simulink model "HSat_orbit"  (R2023a)
settings: Solver=FixedStepAuto  StartTime=0  StopTime=86400*900  MaxStep=3600  RelTol=1e-3  EnableMultiTasking=on
values from neighbouring files (symbols this model uses):
  ext_ENV_G = 6.674e-11    [HSat_op_setup.m]    (also in HSat_op_setup_merged_maria.m)
  ext_ENV_muEarth = 3.986005e14    (= 398600500000000)    [GEO_insertion_setup.m]    (also in HSat_op_setup.m; HSat_op_setup_merged_maria.m; init_orbit_analysis_with_drag_loss.m)
  ext_ENV_Re = 6.37813700*10^6    (= 6378137)    [HSat_op_setup.m]    (also in HSat_op_setup_merged_maria.m)
  ext_EOR_atmosphere_end = 1000e3    (= 1000000)    [HSat_op_setup.m]    (also in HSat_op_setup_merged_maria.m)
  ext_EOR_perigeeraise_end = 600e3    (= 600000)    [HSat_op_setup.m]    (also in HSat_op_setup_merged_maria.m)
  ext_Main_initDate_IC_T = sim_start    [HSat_op_setup.m]    (also in HSat_op_setup_merged_maria.m)
  ext_SC_activecorr_COE_ECI = [1, 1, 1, 0, 0, 0, 0, 0 ]    [HSat_op_setup.m]    (also in HSat_op_setup_merged_maria.m)
  ext_SC_balanced_COE_ECI = [ .500    0.70    1.100 1 1]    [HSat_op_setup.m]    (also in HSat_op_setup_merged_maria.m = [ 0.10 2.10 1.40    1.0000    1.0000]; launch_settings.m)
  ext_SC_cutofferror_COE_ECI = [150e3, .01, 0.1*pi/180, .1*pi/180,.1*pi/180, 0, 0, 0]    [HSat_op_setup.m]    (also in HSat_op_setup_merged_maria.m)
  ext_SC_init_COE_ECI = [a0,ecc0,i0,an0,ap0,tran0,eccan0,ma0]    [HSat_op_setup.m]    (also in HSat_op_setup_merged_maria.m)
  ext_SC_target_COE_ECI = [a1,ecc1,i1,an1,ap1,tran1,eccan1,ma1]    [HSat_op_setup.m]    (also in HSat_op_setup_merged_maria.m)
  ext_SC_target_lambda = 67*pi/180    (= 1.16937059884)    [HSat_op_setup.m]    (also in HSat_op_setup_merged_maria.m)
  sim_SC_init_CoG_EOR_dry = [-0.00448 0.00106 0.46931]    [HSat_op_setup.m]    (also in HSat_op_setup_merged_maria.m)
  sim_SC_init_CoG_propellant = [0 0 0.24758]    [HSat_op_setup.m]    (also in HSat_op_setup_merged_maria.m)
  sim_SC_init_dry_mass = sim_SC_init_wet_mass-sim_SC_init_propellant_mass    (= 727)    [HSat_op_setup.m]    (also in HSat_op_setup_merged_maria.m = 813.7)
  sim_SC_init_wet_mass = 750    [HSat_op_setup.m]    (also in HSat_op_setup_merged_maria.m)
  sim_thrust_force = [ ... (first row only)    [HSat_op_setup.m]    (also in HSat_op_setup_merged_maria.m)
  sim_thrust_massflow = [ ... (first row only)    [HSat_op_setup.m]    (also in HSat_op_setup_merged_maria.m)
  sim_thrust_vector = [ ... (first row only)    [HSat_op_setup.m]    (also in HSat_op_setup_merged_maria.m)
  sim_thruster_position = [ ... (first row only)    [HSat_op_setup.m]    (also in HSat_op_setup_merged_maria.m)
  sim_ts_save = 60    [HSat_op_setup.m]    (also in HSat_op_setup_merged_maria.m)
  third_body_jupiter = 1    [HSat_op_setup.m]    (also in HSat_op_setup_merged_maria.m)
  third_body_moon = 1    [HSat_op_setup.m]    (also in HSat_op_setup_merged_maria.m)
  third_body_sun = 1    [HSat_op_setup.m]    (also in HSat_op_setup_merged_maria.m)
libraries: aerolibutil x26, simulink x12, sharedtransform x7, sharedutil x4, Toolbox x3, matrix_library x1, simulink_extras x1
(part 3 of 5)

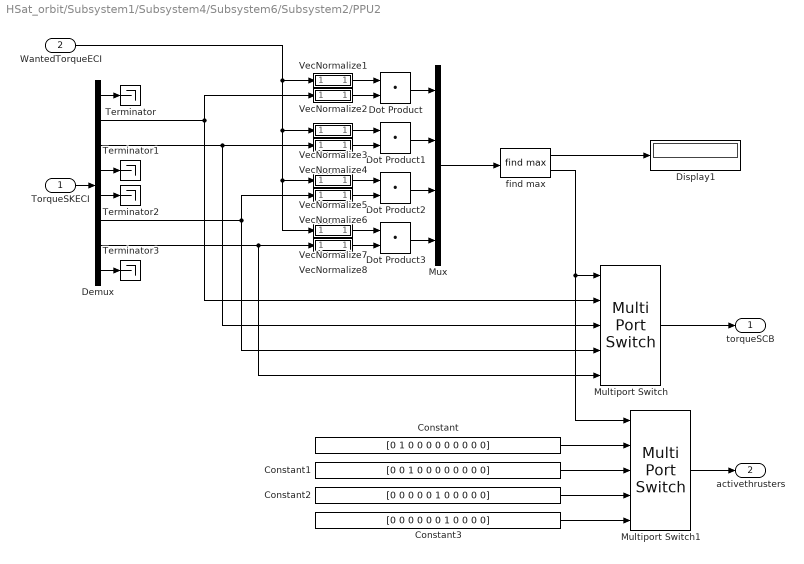
== system HSat_orbit/Subsystem1/Subsystem4/Subsystem6/Subsystem2/PPU2 ==
  TorqueSKECI : Inport
  WantedTorqueECI : Inport  Port=2
  Constant : Constant  Value=[0 1 0 0 0 0 0 0 0 0 0]
  Constant1 : Constant  Value=[0 0 1 0 0 0 0 0 0 0 0]
  Constant2 : Constant  Value=[0 0 0 0 0 1 0 0 0 0 0]
  Constant3 : Constant  Value=[0 0 0 0 0 0 1 0 0 0 0]
  Demux : Demux  Outputs=8
  Display1 : Display
  Dot Product{,1..3} (4 alike) : DotProduct  OutDataTypeStr=Inherit: Inherit via internal rule
  Multiport Switch : MultiPortSwitch  Inputs=4  SaturateOnIntegerOverflow=off  InputSameDT=off
  Multiport Switch1 : MultiPortSwitch  Inputs=4  SaturateOnIntegerOverflow=off  InputSameDT=off
  Mux : Mux
  Terminator{,1..3} (4 alike) : Terminator
  VecNormalize1 : Subsystem
      mask Display: disp('u/||u||')
  VecNormalize2 : Subsystem
      mask Display: disp('u/||u||')
  VecNormalize3 : Subsystem
      mask Display: disp('u/||u||')
  VecNormalize4 : Subsystem
      mask Display: disp('u/||u||')
  VecNormalize5 : Subsystem
      mask Display: disp('u/||u||')
  VecNormalize6 : Subsystem
      mask Display: disp('u/||u||')
  VecNormalize7 : Subsystem
      mask Display: disp('u/||u||')
  VecNormalize8 : Subsystem
      mask Display: disp('u/||u||')
  find max : Toolbox/vector blocks/find max  SystemSampleTime=-1  VariantActivationTime=update diagram  Latency=0  AutoFrameSizeCalculation=off
      settings: SourceProductName=SSC flight toolbox
  torqueSCB : Outport
  activethrusters : Outport  Port=2
  wires:
  TorqueSKECI/1 -> Demux/1
  Demux/2 -> VecNormalize2/1(In1), Multiport Switch/2
  Demux/3 -> Multiport Switch/3, VecNormalize4/1(In1)
  Demux/6 -> VecNormalize6/1(In1), Multiport Switch/4
  Demux/7 -> Multiport Switch/5, VecNormalize8/1(In1)
  WantedTorqueECI/1 -> VecNormalize1/1(In1), VecNormalize3/1(In1), VecNormalize5/1(In1), VecNormalize7/1(In1)
  VecNormalize1/1(Out1) -> Dot Product/1
  VecNormalize2/1(Out1) -> Dot Product/2
  VecNormalize3/1(Out1) -> Dot Product1/1
  VecNormalize4/1(Out1) -> Dot Product1/2
  VecNormalize5/1(Out1) -> Dot Product2/1
  VecNormalize6/1(Out1) -> Dot Product2/2
  VecNormalize7/1(Out1) -> Dot Product3/1
  VecNormalize8/1(Out1) -> Dot Product3/2
  Dot Product/1 -> Mux/1
  Dot Product1/1 -> Mux/2
  Dot Product2/1 -> Mux/3
  Dot Product3/1 -> Mux/4
  Mux/1 -> find max/1
  find max/1 -> Display1/1
  Multiport Switch/1 -> torqueSCB/1
  Demux/5 -> Terminator2/1
  Demux/4 -> Terminator1/1
  Demux/1 -> Terminator/1
  Demux/8 -> Terminator3/1
  Multiport Switch1/1 -> activethrusters/1
  Constant/1 -> Multiport Switch1/2
  Constant1/1 -> Multiport Switch1/3
  Constant3/1 -> Multiport Switch1/5
  find max/2 -> Multiport Switch1/1, Multiport Switch/1
  Constant2/1 -> Multiport Switch1/4

== system HSat_orbit/Subsystem1/Subsystem4/Subsystem6/Subsystem2/Subsystem ==
  AllTorquesSCB : Inport
  q_eci2scb_wanted : Inport  Port=2
  Mux : Mux  Inputs=8
  Quaternion Rotation{,1..7} (8 alike) : aerolibutil/Quaternion Rotation
  TorqueSCBSK1 : Selector  NumberOfDimensions=2  InputPortWidth=3  IndexOptions=Index vector (dialog),Index vector (dialog)  Indices=1,[1 2 3]  OutputSizes=1,1
  TorqueSCBSK2 : Selector  NumberOfDimensions=2  InputPortWidth=3  IndexOptions=Index vector (dialog),Index vector (dialog)  Indices=2,[1 2 3]  OutputSizes=1,1
  TorqueSCBSK3 : Selector  NumberOfDimensions=2  InputPortWidth=3  IndexOptions=Index vector (dialog),Index vector (dialog)  Indices=3,[1 2 3]  OutputSizes=1,1
  TorqueSCBSK4 : Selector  NumberOfDimensions=2  InputPortWidth=3  IndexOptions=Index vector (dialog),Index vector (dialog)  Indices=4,[1 2 3]  OutputSizes=1,1
  TorqueSCBSK5 : Selector  NumberOfDimensions=2  InputPortWidth=3  IndexOptions=Index vector (dialog),Index vector (dialog)  Indices=5,[1 2 3]  OutputSizes=1,1
  TorqueSCBSK6 : Selector  NumberOfDimensions=2  InputPortWidth=3  IndexOptions=Index vector (dialog),Index vector (dialog)  Indices=6,[1 2 3]  OutputSizes=1,1
  TorqueSCBSK7 : Selector  NumberOfDimensions=2  InputPortWidth=3  IndexOptions=Index vector (dialog),Index vector (dialog)  Indices=7,[1 2 3]  OutputSizes=1,1
  TorqueSCBSK8 : Selector  NumberOfDimensions=2  InputPortWidth=3  IndexOptions=Index vector (dialog),Index vector (dialog)  Indices=8,[1 2 3]  OutputSizes=1,1
  TorqueSKECI : Outport
  wires:
  TorqueSCBSK5/1 -> Quaternion Rotation4/2
  Quaternion Rotation3/1 -> Mux/4  "TorqueECISK4"
  Quaternion Rotation6/1 -> Mux/7  "TorqueECISK7"
  Quaternion Rotation4/1 -> Mux/5  "TorqueECISK5"
  TorqueSCBSK3/1 -> Quaternion Rotation2/2
  Quaternion Rotation/1 -> Mux/1  "TorqueECISK1"
  Quaternion Rotation7/1 -> Mux/8  "TorqueECISK8"
  TorqueSCBSK2/1 -> Quaternion Rotation1/2
  Quaternion Rotation2/1 -> Mux/3  "TorqueECISK3"
  TorqueSCBSK4/1 -> Quaternion Rotation3/2
  q_eci2scb_wanted/1 -> Quaternion Rotation7/1, Quaternion Rotation6/1, Quaternion Rotation5/1, Quaternion Rotation4/1, Quaternion Rotation3/1, Quaternion Rotation2/1, Quaternion Rotation1/1, Quaternion Rotation/1
  TorqueSCBSK8/1 -> Quaternion Rotation7/2
  TorqueSCBSK7/1 -> Quaternion Rotation6/2
  TorqueSCBSK1/1 -> Quaternion Rotation/2
  Quaternion Rotation5/1 -> Mux/6  "TorqueECISK6"
  TorqueSCBSK6/1 -> Quaternion Rotation5/2
  AllTorquesSCB/1 -> TorqueSCBSK8/1, TorqueSCBSK7/1, TorqueSCBSK6/1, TorqueSCBSK5/1, TorqueSCBSK4/1, TorqueSCBSK3/1, TorqueSCBSK2/1, TorqueSCBSK1/1
  Quaternion Rotation1/1 -> Mux/2  "TorqueECISK2"
  Mux/1 -> TorqueSKECI/1

== system HSat_orbit/Subsystem1/Subsystem4/Subsystem6/Subsystem2/Subsystem1 ==
  TorqueSCB : Inport
  WantedTorqueECI : Inport  Port=2
  sunvECI : Inport  Port=3
  Quaternion Multiplication : aerolibutil/Quaternion Multiplication
  Subsystem : Subsystem
  q_scb_calc : Subsystem
  q_eci2scb : Outport
  wires:
  Quaternion Multiplication/1 -> q_eci2scb/1
  sunvECI/1 -> q_scb_calc/2(sunvECI)
  q_scb_calc/1(qECI2scbp) -> Quaternion Multiplication/1
  TorqueSCB/1 -> Subsystem/1(EORthrustSCB)
  Subsystem/1(qscbp2scb) -> Quaternion Multiplication/2
  WantedTorqueECI/1 -> q_scb_calc/1(torqueECI)  "vec_eci"

== system HSat_orbit/Subsystem1/Dynamics/Subsystem/3 body perturbation legendre polynomial/Subsystem1/cos angle ==
  sat : Inport
  3 body : Inport  Port=2
  Divide : Product  Inputs=*//
  Dot Product : DotProduct  OutDataTypeStr=Inherit: Inherit via internal rule
  Dot Product1 : DotProduct  OutDataTypeStr=Inherit: Inherit via internal rule
  Dot Product2 : DotProduct  OutDataTypeStr=Inherit: Inherit via internal rule
  Sqrt : Sqrt
  Sqrt1 : Sqrt
  cos angle : Outport
  wires:
  3 body/1 -> Dot Product1/2, Dot Product1/1, Dot Product/2
  Dot Product1/1 -> Sqrt/1
  sat/1 -> Dot Product/1, Dot Product2/1, Dot Product2/2
  Dot Product2/1 -> Sqrt1/1
  Dot Product/1 -> Divide/1
  Sqrt/1 -> Divide/3
  Sqrt1/1 -> Divide/2
  Divide/1 -> cos angle/1

== system HSat_orbit/Subsystem1/Dynamics/Subsystem/3 body perturbation legendre polynomial/Subsystem2/cos angle ==
  sat : Inport
  3 body : Inport  Port=2
  Divide : Product  Inputs=*//
  Dot Product : DotProduct  OutDataTypeStr=Inherit: Inherit via internal rule
  Dot Product1 : DotProduct  OutDataTypeStr=Inherit: Inherit via internal rule
  Dot Product2 : DotProduct  OutDataTypeStr=Inherit: Inherit via internal rule
  Sqrt : Sqrt
  Sqrt1 : Sqrt
  cos angle : Outport
  wires:
  3 body/1 -> Dot Product1/2, Dot Product1/1, Dot Product/2
  Dot Product1/1 -> Sqrt/1
  sat/1 -> Dot Product/1, Dot Product2/1, Dot Product2/2
  Dot Product2/1 -> Sqrt1/1
  Dot Product/1 -> Divide/1
  Sqrt/1 -> Divide/3
  Sqrt1/1 -> Divide/2
  Divide/1 -> cos angle/1

== system HSat_orbit/Subsystem1/Dynamics/Subsystem/3 body perturbation legendre polynomial/Subsystem3/cos angle ==
  sat : Inport
  3 body : Inport  Port=2
  Divide : Product  Inputs=*//
  Dot Product : DotProduct  OutDataTypeStr=Inherit: Inherit via internal rule
  Dot Product1 : DotProduct  OutDataTypeStr=Inherit: Inherit via internal rule
  Dot Product2 : DotProduct  OutDataTypeStr=Inherit: Inherit via internal rule
  Sqrt : Sqrt
  Sqrt1 : Sqrt
  cos angle : Outport
  wires:
  3 body/1 -> Dot Product1/2, Dot Product1/1, Dot Product/2
  Dot Product1/1 -> Sqrt/1
  sat/1 -> Dot Product/1, Dot Product2/1, Dot Product2/2
  Dot Product2/1 -> Sqrt1/1
  Dot Product/1 -> Divide/1
  Sqrt/1 -> Divide/3
  Sqrt1/1 -> Divide/2
  Divide/1 -> cos angle/1

== system HSat_orbit/Subsystem1/Navigation/Subsystem/Subsystem2/Subsystem1/Norm3 ==
  In1 : Inport
  Dot Product : DotProduct  OutDataTypeStr=Inherit: Inherit via internal rule
  Sqrt : Sqrt
  Out1 : Outport
  wires:
  In1/1 -> Dot Product/1, Dot Product/2
  Sqrt/1 -> Out1/1
  Dot Product/1 -> Sqrt/1

== system HSat_orbit/Subsystem1/Navigation/Subsystem/Subsystem2/Subsystem1/Subsystem ==
  lambda : Inport
  Constant2 : Constant  Value=2*pi
  Constant3 : Constant  Value=pi
  Math Function2 : Math  Operator=mod
  Sum10 : Sum  Inputs=|+-
  Sum9 : Sum  Inputs=|++
  Out1 : Outport
  wires:
  lambda/1 -> Sum9/1
  Sum9/1 -> Math Function2/1
  Constant3/1 -> Sum9/2, Sum10/2
  Math Function2/1 -> Sum10/1
  Sum10/1 -> Out1/1
  Constant2/1 -> Math Function2/2

== system HSat_orbit/Subsystem1/Navigation/Subsystem/Subsystem2/Subsystem1/Subsystem1 ==
  lambda : Inport
  Constant4 : Constant  Value=2*pi
  Constant5 : Constant  Value=pi
  Math Function3 : Math  Operator=mod
  Sum11 : Sum  Inputs=|+-
  Sum12 : Sum  Inputs=|++
  Out1 : Outport
  wires:
  Sum11/1 -> Out1/1
  lambda/1 -> Sum12/1
  Sum12/1 -> Math Function3/1
  Math Function3/1 -> Sum11/1
  Constant5/1 -> Sum12/2, Sum11/2
  Constant4/1 -> Math Function3/2

== system HSat_orbit/Subsystem1/Navigation/Subsystem/Subsystem2/Subsystem1/Subsystem2 ==
  a : Inport
  Constant1 : Constant  Value=ext_ENV_muEarth
  Constant2 : Constant  Value=3
  Constant4 : Constant
  Divide : Product  Inputs=*/
  Gain : Gain  Gain=2*pi
  Gain1 : Gain  Gain=2*pi
  Gain3 : Gain
  Gain4 : Gain  Gain=1/86400
  Math Function : Math  Operator=pow
  Math Function1 : Math  Operator=reciprocal
  Sqrt : Sqrt
  Subtract : Sum  Inputs=+-
  lambdadot : Outport
  wires:
  Subtract/1 -> Gain1/1  "lambdadot"
  Constant4/1 -> Subtract/2
  Constant2/1 -> Math Function/2
  Sqrt/1 -> Gain/1
  Math Function/1 -> Divide/1
  Constant1/1 -> Divide/2
  Math Function1/1 -> Gain3/1
  a/1 -> Math Function/1
  Divide/1 -> Sqrt/1
  Gain1/1 -> lambdadot/1
  Gain/1 -> Gain4/1
  Gain3/1 -> Subtract/1
  Gain4/1 -> Math Function1/1

== system HSat_orbit/Subsystem1/Navigation/Subsystem/Subsystem2/Subsystem1/Subsystem3 ==
  lambda : Inport
  Constant6 : Constant  Value=2*pi
  Constant7 : Constant  Value=pi
  Math Function4 : Math  Operator=mod
  Sum13 : Sum  Inputs=|+-
  Sum14 : Sum  Inputs=|++
  Out1 : Outport
  wires:
  Sum14/1 -> Math Function4/1
  Constant6/1 -> Math Function4/2
  Math Function4/1 -> Sum13/1
  Sum13/1 -> Out1/1
  lambda/1 -> Sum14/1
  Constant7/1 -> Sum14/2, Sum13/2

== system HSat_orbit/Subsystem1/Navigation/Subsystem/Subsystem2/Subsystem7/Norm1 ==
  In1 : Inport
  Dot Product : DotProduct  OutDataTypeStr=Inherit: Inherit via internal rule
  Sqrt : Sqrt
  Out1 : Outport
  wires:
  In1/1 -> Dot Product/1, Dot Product/2
  Sqrt/1 -> Out1/1
  Dot Product/1 -> Sqrt/1

== system HSat_orbit/Subsystem1/Navigation/Subsystem/Subsystem2/Subsystem7/Norm2 ==
  In1 : Inport
  Dot Product : DotProduct  OutDataTypeStr=Inherit: Inherit via internal rule
  Sqrt : Sqrt
  Out1 : Outport
  wires:
  In1/1 -> Dot Product/1, Dot Product/2
  Sqrt/1 -> Out1/1
  Dot Product/1 -> Sqrt/1

== system HSat_orbit/Subsystem1/Navigation/Subsystem/Subsystem2/Subsystem7/Subsystem ==
  r : Inport
  rabs : Inport  Port=2
  v : Inport  Port=3
  Divide : Product  Inputs=*/
  Dot Product : DotProduct  OutDataTypeStr=Inherit: Inherit via internal rule
  Dot Product1 : DotProduct  OutDataTypeStr=Inherit: Inherit via internal rule
  Math Function : Math  Operator=square
  Sqrt : Sqrt
  Subtract1 : Sum  Inputs=+-
  vr : Outport
  vp : Outport  Port=2
  wires:
  Sqrt/1 -> vp/1  "vp"
  rabs/1 -> Divide/2
  Subtract1/1 -> Sqrt/1
  r/1 -> Divide/1
  Dot Product1/1 -> Subtract1/1  "vr"
  Divide/1 -> Dot Product/1
  Math Function/1 -> Subtract1/2
  v/1 -> Dot Product/2, Dot Product1/1, Dot Product1/2
  Dot Product/1 -> vr/1, Math Function/1  "vr"

== system HSat_orbit/Subsystem1/Navigation/Subsystem/Subsystem2/Subsystem7/Subsystem1 ==
  h : Inport
  Constant : Constant  Value=0
  Divide2 : Product  Inputs=*/
  Mux : Mux  Inputs=3
  Norm4 : Subsystem  Tag=||u||
      mask Display: disp('||u||')
  Selector1 : Selector  InputPortWidth=3  IndexOptions=Index vector (dialog)  Indices=[2]  OutputSizes=1
  Selector2 : Selector  InputPortWidth=3  IndexOptions=Index vector (dialog)  Indices=[1]  OutputSizes=1
  Selector3 : Selector  InputPortWidth=3  IndexOptions=Index vector (dialog)  Indices=[1]  OutputSizes=1
  Trigonometric Function1 : Trigonometry  Operator=acos
  Unary Minus : UnaryMinus
  N : Outport
  N_abs : Outport  Port=2
  Raan : Outport  Port=3
  wires:
  Trigonometric Function1/1 -> Raan/1  "Raan"
  Unary Minus/1 -> Mux/1
  Selector1/1 -> Unary Minus/1
  Divide2/1 -> Trigonometric Function1/1
  Norm4/1(Out1) -> Divide2/2, N_abs/1  "N_abs"
  Constant/1 -> Mux/3
  Selector3/1 -> Divide2/1
  Selector2/1 -> Mux/2
  h/1 -> Selector2/1, Selector1/1
  Mux/1 -> N/1, Selector3/1, Norm4/1(In1)  "N"

== system HSat_orbit/Subsystem1/Navigation/Subsystem/Subsystem2/Subsystem7/Subsystem2 ==
  h : Inport
  Divide1 : Product  Inputs=*/
  Norm3 : Subsystem  Tag=||u||
      mask Display: disp('||u||')
  Selector : Selector  InputPortWidth=3  IndexOptions=Index vector (dialog)  Indices=[3]  OutputSizes=1
  Trigonometric Function : Trigonometry  Operator=acos
  i : Outport
  wires:
  Trigonometric Function/1 -> i/1  "i"
  Selector/1 -> Divide1/1
  h/1 -> Norm3/1(In1), Selector/1
  Norm3/1(Out1) -> Divide1/2
  Divide1/1 -> Trigonometric Function/1

== system HSat_orbit/Subsystem1/Navigation/Subsystem/Subsystem2/Subsystem7/Subsystem3 ==
  r : Inport
  rabs : Inport  Port=2
  v : Inport  Port=3
  vabs : Inport  Port=4
  Constant1 : Constant  Value=ext_ENV_muEarth
  Constant3 : Constant
  Divide3 : Product  Inputs=*/
  Divide4 : Product  Inputs=*/
  Divide5 : Product  Inputs=**
  Divide6 : Product  Inputs=**
  Divide7 : Product  Inputs=**
  Dot Product : DotProduct  OutDataTypeStr=Inherit: Inherit via internal rule
  Math Function1 : Math  Operator=square
  Norm5 : Subsystem  Tag=||u||
      mask Display: disp('||u||')
  Subtract : Sum  Inputs=-+
  Subtract1 : Sum  Inputs=+-
  e_vec : Outport
  e_abs : Outport  Port=2
  wires:
  rabs/1 -> Divide4/2
  r/1 -> Dot Product/1, Divide5/1
  Subtract1/1 -> Divide7/2
  Norm5/1(Out1) -> e_abs/1  "e_abs"
  Divide7/1 -> Norm5/1(In1), e_vec/1  "e"
  Constant3/1 -> Divide3/1
  vabs/1 -> Math Function1/1
  Constant1/1 -> Divide4/1, Divide3/2
  Subtract/1 -> Divide5/2
  Divide5/1 -> Subtract1/1
  Divide4/1 -> Subtract/1
  v/1 -> Dot Product/2, Divide6/2
  Divide6/1 -> Subtract1/2
  Dot Product/1 -> Divide6/1
  Math Function1/1 -> Subtract/2
  Divide3/1 -> Divide7/1

== system HSat_orbit/Subsystem1/Navigation/Subsystem/Subsystem2/Subsystem7/Subsystem4 ==
  e : Inport
  eabs : Inport  Port=2
  N : Inport  Port=3
  Nabs : Inport  Port=4
  Divide8 : Product  Inputs=*/
  Divide9 : Product  Inputs=**
  Dot Product1 : DotProduct  OutDataTypeStr=Inherit: Inherit via internal rule
  Trigonometric Function2 : Trigonometry  Operator=acos
  argp : Outport
  wires:
  Nabs/1 -> Divide9/2
  N/1 -> Dot Product1/2
  Divide9/1 -> Divide8/2  "e"
  Trigonometric Function2/1 -> argp/1  "argp"
  Dot Product1/1 -> Divide8/1
  e/1 -> Dot Product1/1
  eabs/1 -> Divide9/1
  Divide8/1 -> Trigonometric Function2/1

== system HSat_orbit/Subsystem1/Navigation/Subsystem/Subsystem2/Subsystem7/Subsystem5 ==
  vr : Inport
  e : Inport  Port=2
  eabs : Inport  Port=3
  r : Inport  Port=4
  rabs : Inport  Port=5
  Constant : Constant  Value=2*pi
  Subsystem : Subsystem
  Subsystem1 : Subsystem
  Subsystem2 : Subsystem
  Subsystem3 : Subsystem
  Subtract : Sum  Inputs=+-
  Switch : Switch  Criteria=u2 > Threshold  SaturateOnIntegerOverflow=off  InputSameDT=off
  nu : Outport
  M : Outport  Port=2
  E : Outport  Port=3
  nu igen : Outport  Port=4
  wires:
  eabs/1 -> Subsystem1/2(eabs), Subsystem3/2(eabs), Subsystem/2(eabs), Subsystem2/3(eabs)  "eabs"
  Subsystem/1(E) -> Subsystem1/1(E), Subsystem3/1(E), E/1  "E"
  Subsystem2/1(nu) -> Switch/1, Subtract/2
  e/1 -> Subsystem2/1(e)
  r/1 -> Subsystem2/2(r)
  rabs/1 -> Subsystem2/4(rabs)
  Subsystem3/1(nu) -> nu igen/1
  vr/1 -> Switch/2
  Switch/1 -> nu/1, Subsystem/1(nu)  "nu"
  Constant/1 -> Subtract/1
  Subtract/1 -> Switch/3
  Subsystem1/1(M) -> M/1  "M"

== system HSat_orbit/Subsystem1/Navigation/Subsystem/Subsystem2/Subsystem7/Subsystem6 ==
  rabs : Inport
  vabs : Inport  Port=2
  Constant3 : Constant
  Constant4 : Constant  Value=2
  Constant5 : Constant  Value=ext_ENV_muEarth
  Divide1 : Product  Inputs=*/
  Divide3 : Product  Inputs=*/
  Divide4 : Product  Inputs=*/
  Math Function1 : Math  Operator=square
  Subtract : Sum  Inputs=+-
  a : Outport
  wires:
  Divide3/1 -> a/1  "a"
  vabs/1 -> Math Function1/1
  Divide4/1 -> Subtract/1
  Math Function1/1 -> Divide1/1
  Constant4/1 -> Divide4/1
  rabs/1 -> Divide4/2
  Divide1/1 -> Subtract/2
  Subtract/1 -> Divide3/2
  Constant3/1 -> Divide3/1
  Constant5/1 -> Divide1/2

== system HSat_orbit/Subsystem1/Subsystem4/EORattitude/Subsystem/Subsystem1/Subsystem ==
  EORthrustSCB : Inport
  Flipsign : Inport  Port=2
  Create 3x3 Matrix : sharedutil/Create 3x3 Matrix  aMode=aMode
      settings: LibrarySourceBlock=aerolibutil/Create 3x3 Matrix
  Demux : Demux  Outputs=3
  Demux1 : Demux  Outputs=3
  Demux2 : Demux  Outputs=3
  Direction Cosine Matrix to Quaternions : sharedtransform/Direction Cosine Matrix  to Quaternions  aMode=0  action=None  tolerance=eps(2)
      settings: LibrarySourceBlock=|
      | aerolibtransform2/Direction Cosine Matrix
      | to Quaternions
  Divide : Product  Inputs=**
  Quaternion Inverse : aerolibutil/Quaternion Inverse
  VecNormalize4 : Subsystem
      mask Display: disp('u/||u||')
  Zeci x Reci : Subsystem  mask(Cross Product){}
      mask help: Calculates the cross product of two 3x1 vectors.
      mask Help:
      | <p>This block calculates the cross product of two 3x1 vectors, ie.</p>
      | 
      | <ul>C(1) = A(2)*B(3) - A(3)*B(2)</ul>
      | <ul>C(2) = A(3)*B(1) - A(1)*B(3)</ul>
      | <ul>C(3) = A(1)*B(2) - A(2)*B(1)</ul>
      | 
      | <p>The block inputs and output contain more than one signal as described below.</p>
      | 
      | <p><H4>Block Vector Input 1 - A</H4>
      | <ul>
      | <li>A(1)</li>
      | <li>A(2)</li>
      | <li>A(3)</li>
      | </ul>
      | </p>
      | 
      | <p><H4>Block Vector Input 2 - B</H4>
      | <ul>
      | <li>B(1)</li>
      | <li>B(2)</li>
      | <li>B(3)</li>
      | </ul>
      | </p>
      | 
      | <p><H4>Block Vector Output - Cross Product (AxB)</H4>
      | <ul>
      | <li>C(1)</li>
      | <li>C(2)</li>
      | <li>C(3)</li>
      | </ul>
      | </p>
      mask Display: disp('Cross\nProduct')
  Zeci x Reci1 : Subsystem  mask(Cross Product){}
      mask help: Calculates the cross product of two 3x1 vectors.
      mask Help:
      | <p>This block calculates the cross product of two 3x1 vectors, ie.</p>
      | 
      | <ul>C(1) = A(2)*B(3) - A(3)*B(2)</ul>
      | <ul>C(2) = A(3)*B(1) - A(1)*B(3)</ul>
      | <ul>C(3) = A(1)*B(2) - A(2)*B(1)</ul>
      | 
      | <p>The block inputs and output contain more than one signal as described below.</p>
      | 
      | <p><H4>Block Vector Input 1 - A</H4>
      | <ul>
      | <li>A(1)</li>
      | <li>A(2)</li>
      | <li>A(3)</li>
      | </ul>
      | </p>
      | 
      | <p><H4>Block Vector Input 2 - B</H4>
      | <ul>
      | <li>B(1)</li>
      | <li>B(2)</li>
      | <li>B(3)</li>
      | </ul>
      | </p>
      | 
      | <p><H4>Block Vector Output - Cross Product (AxB)</H4>
      | <ul>
      | <li>C(1)</li>
      | <li>C(2)</li>
      | <li>C(3)</li>
      | </ul>
      | </p>
      mask Display: disp('Cross\nProduct')
  yscbSCB : Constant  Value=[0 1 0]
  qscbp2scb : Outport
  wires:
  Direction Cosine Matrix to Quaternions/1 -> Quaternion Inverse/1  "qscbp2scb"
  Flipsign/1 -> Divide/1
  Demux2/3 -> Create 3x3 Matrix/9
  Demux2/1 -> Create 3x3 Matrix/7
  Demux/1 -> Create 3x3 Matrix/1
  Demux1/2 -> Create 3x3 Matrix/5
  EORthrustSCB/1 -> VecNormalize4/1(In1)
  Demux2/2 -> Create 3x3 Matrix/8
  Demux/3 -> Create 3x3 Matrix/3
  yscbSCB/1 -> Divide/2
  Zeci x Reci/1(c(1) c(2) c(3)) -> Zeci x Reci1/2(b(1) b(2) b(3)), Demux/1  "xscbpSCB"
  Demux/2 -> Create 3x3 Matrix/2
  Create 3x3 Matrix/1 -> Direction Cosine Matrix to Quaternions/1
  Zeci x Reci1/1(c(1) c(2) c(3)) -> Demux1/1  "yscbpSCB"
  Demux1/3 -> Create 3x3 Matrix/6
  Demux1/1 -> Create 3x3 Matrix/4
  Divide/1 -> Zeci x Reci/1(a(1) a(2) a(3))
  VecNormalize4/1(Out1) -> Demux2/1, Zeci x Reci1/1(a(1) a(2) a(3)), Zeci x Reci/2(b(1) b(2) b(3))  "zscbpSCB"
  Quaternion Inverse/1 -> qscbp2scb/1

== system HSat_orbit/Subsystem1/Subsystem4/EORattitude/Subsystem/Subsystem1/q_scb_calc ==
  EORthrustECI : Inport
  sunvECI : Inport  Port=2
  Direction Cosine Matrix to Quaternions : sharedtransform/Direction Cosine Matrix  to Quaternions  aMode=0  action=None  tolerance=eps(2)
      settings: LibrarySourceBlock=|
      | aerolibtransform2/Direction Cosine Matrix
      | to Quaternions
  Matrix Concatenate : Concatenate  NumInputs=3  Mode=Multidimensional array
  Reshape1 : Reshape  OutputDimensionality=Row vector (2-D)
  Reshape2 : Reshape  OutputDimensionality=Row vector (2-D)
  Reshape3 : Reshape  OutputDimensionality=Row vector (2-D)
  VecNormalize : Subsystem
      mask Display: disp('u/||u||')
  VecNormalize1 : Subsystem
      mask Display: disp('u/||u||')
  VecNormalize2 : Subsystem
      mask Display: disp('u/||u||')
  VecNormalize3 : Subsystem
      mask Display: disp('u/||u||')
  Yscb x Zscb : Subsystem  mask(Cross Product){}
      mask help: Calculates the cross product of two 3x1 vectors.
      mask Help:
      | <p>This block calculates the cross product of two 3x1 vectors, ie.</p>
      | 
      | <ul>C(1) = A(2)*B(3) - A(3)*B(2)</ul>
      | <ul>C(2) = A(3)*B(1) - A(1)*B(3)</ul>
      | <ul>C(3) = A(1)*B(2) - A(2)*B(1)</ul>
      | 
      | <p>The block inputs and output contain more than one signal as described below.</p>
      | 
      | <p><H4>Block Vector Input 1 - A</H4>
      | <ul>
      | <li>A(1)</li>
      | <li>A(2)</li>
      | <li>A(3)</li>
      | </ul>
      | </p>
      | 
      | <p><H4>Block Vector Input 2 - B</H4>
      | <ul>
      | <li>B(1)</li>
      | <li>B(2)</li>
      | <li>B(3)</li>
      | </ul>
      | </p>
      | 
      | <p><H4>Block Vector Output - Cross Product (AxB)</H4>
      | <ul>
      | <li>C(1)</li>
      | <li>C(2)</li>
      | <li>C(3)</li>
      | </ul>
      | </p>
      mask Display: disp('Cross\nProduct')
  Zeci x Reci : Subsystem  mask(Cross Product){}
      mask help: Calculates the cross product of two 3x1 vectors.
      mask Help:
      | <p>This block calculates the cross product of two 3x1 vectors, ie.</p>
      | 
      | <ul>C(1) = A(2)*B(3) - A(3)*B(2)</ul>
      | <ul>C(2) = A(3)*B(1) - A(1)*B(3)</ul>
      | <ul>C(3) = A(1)*B(2) - A(2)*B(1)</ul>
      | 
      | <p>The block inputs and output contain more than one signal as described below.</p>
      | 
      | <p><H4>Block Vector Input 1 - A</H4>
      | <ul>
      | <li>A(1)</li>
      | <li>A(2)</li>
      | <li>A(3)</li>
      | </ul>
      | </p>
      | 
      | <p><H4>Block Vector Input 2 - B</H4>
      | <ul>
      | <li>B(1)</li>
      | <li>B(2)</li>
      | <li>B(3)</li>
      | </ul>
      | </p>
      | 
      | <p><H4>Block Vector Output - Cross Product (AxB)</H4>
      | <ul>
      | <li>C(1)</li>
      | <li>C(2)</li>
      | <li>C(3)</li>
      | </ul>
      | </p>
      mask Display: disp('Cross\nProduct')
  qECI2scbp : Outport  InitialOutput=0
  wires:
  Zeci x Reci/1(c(1) c(2) c(3)) -> VecNormalize3/1(In1)  "Y"
  VecNormalize1/1(Out1) -> Yscb x Zscb/2(b(1) b(2) b(3)), Reshape3/1, Zeci x Reci/2(b(1) b(2) b(3))  "Zscbp"
  Direction Cosine Matrix to Quaternions/1 -> qECI2scbp/1
  EORthrustECI/1 -> VecNormalize1/1(In1)
  VecNormalize3/1(Out1) -> Reshape1/1, Yscb x Zscb/1(a(1) a(2) a(3))  "Yscbp"
  Yscb x Zscb/1(c(1) c(2) c(3)) -> VecNormalize/1(In1)
  sunvECI/1 -> VecNormalize2/1(In1)
  Reshape1/1 -> Matrix Concatenate/2
  Reshape3/1 -> Matrix Concatenate/3
  Reshape2/1 -> Matrix Concatenate/1
  VecNormalize/1(Out1) -> Reshape2/1  "Xscbp"
  VecNormalize2/1(Out1) -> Zeci x Reci/1(a(1) a(2) a(3))
  Matrix Concatenate/1 -> Direction Cosine Matrix to Quaternions/1

== system HSat_orbit/Subsystem1/Subsystem4/EORattitude/Subsystem/Subsystem3/FlipSatellite ==
  AmomSCB : Inport
  EORtorqueSCB : Inport  Port=2
  Compare To Constant : simulink/Logic and Bit Operations/Compare To Constant  relop=>  const=sin((180-70.53)/2*pi/180)*22.5*.75  OutDataTypeStr=boolean
  Compare To Constant1 : simulink/Logic and Bit Operations/Compare To Constant  relop=>  const=cos(80*pi/180)  OutDataTypeStr=boolean
  Compare To Constant2 : simulink/Logic and Bit Operations/Compare To Constant  relop=>  const=sin((180-70.53)/2*pi/180)*22.5*.9  OutDataTypeStr=boolean
  Compare To Constant3 : simulink/Logic and Bit Operations/Compare To Constant  relop=>  const=cos(90*pi/180)  OutDataTypeStr=boolean
  Dot Product : DotProduct  OutDataTypeStr=Inherit: Inherit via internal rule
  Dot Product1 : DotProduct  OutDataTypeStr=Inherit: Inherit via internal rule
  Logical Operator : Logic  AllPortsSameDT=off  OutDataTypeStr=boolean
  Logical Operator1 : Logic  AllPortsSameDT=off  OutDataTypeStr=boolean
  Logical Operator2 : Logic  Operator=OR  AllPortsSameDT=off  OutDataTypeStr=boolean
  Logical Operator3 : Logic  Operator=NOT  AllPortsSameDT=off  OutDataTypeStr=boolean
  Reshape1 : Reshape  OutputDimensionality=Row vector (2-D)
  VecNormalize : Subsystem
      mask Display: disp('u/||u||')
  VecNormalize1 : Subsystem
      mask Display: disp('u/||u||')
  FlipSatellite_bool : Outport
  DoAMOM : Outport  Port=2
  NoAMOM : Outport  Port=3
  wires:
  Logical Operator/1 -> Logical Operator2/1
  EORtorqueSCB/1 -> VecNormalize1/1(In1)
  Dot Product/1 -> Compare To Constant2/1, Compare To Constant/1
  Compare To Constant/1 -> Logical Operator/1
  Dot Product1/1 -> Compare To Constant3/1, Compare To Constant1/1
  Compare To Constant1/1 -> Logical Operator/2
  VecNormalize/1(Out1) -> Dot Product/2, Dot Product1/1
  VecNormalize1/1(Out1) -> Dot Product1/2
  Compare To Constant2/1 -> Logical Operator1/1
  Logical Operator1/1 -> DoAMOM/1, Logical Operator2/2
  Logical Operator2/1 -> FlipSatellite_bool/1
  AmomSCB/1 -> Reshape1/1
  Reshape1/1 -> Dot Product/1, VecNormalize/1(In1)
  Compare To Constant3/1 -> Logical Operator3/1, Logical Operator1/2
  Logical Operator3/1 -> NoAMOM/1

== system HSat_orbit/Subsystem1/Subsystem4/EORattitude/Subsystem/Subsystem3/Subsystem ==
  note: FlipSign
  FlipNow : Inport
  Switch : Switch  Criteria=u2 > Threshold  SaturateOnIntegerOverflow=off
  Unary Minus : UnaryMinus
  Unit Delay : UnitDelay  InitialCondition=1  SampleTime=-1  HasFrameUpgradeWarning=on
  FlipPlusMinus : Outport
  wires:
  FlipNow/1 -> Switch/2
  Unary Minus/1 -> Switch/1
  Switch/1 -> Unit Delay/1
  Unit Delay/1 -> Unary Minus/1, Switch/3, FlipPlusMinus/1

== system HSat_orbit/Subsystem1/Subsystem4/EORattitude/Subsystem4/Subsystem1/Subsystem ==
  EORthrustSCB : Inport
  Create 3x3 Matrix : sharedutil/Create 3x3 Matrix  aMode=aMode
      settings: LibrarySourceBlock=aerolibutil/Create 3x3 Matrix
  Demux : Demux  Outputs=3
  Demux1 : Demux  Outputs=3
  Demux2 : Demux  Outputs=3
  Direction Cosine Matrix to Quaternions : sharedtransform/Direction Cosine Matrix  to Quaternions  aMode=0  action=None  tolerance=eps(2)
      settings: LibrarySourceBlock=|
      | aerolibtransform2/Direction Cosine Matrix
      | to Quaternions
  Quaternion Inverse : aerolibutil/Quaternion Inverse
  VecNormalize4 : Subsystem
      mask Display: disp('u/||u||')
  Zeci x Reci : Subsystem  mask(Cross Product){}
      mask help: Calculates the cross product of two 3x1 vectors.
      mask Help:
      | <p>This block calculates the cross product of two 3x1 vectors, ie.</p>
      | 
      | <ul>C(1) = A(2)*B(3) - A(3)*B(2)</ul>
      | <ul>C(2) = A(3)*B(1) - A(1)*B(3)</ul>
      | <ul>C(3) = A(1)*B(2) - A(2)*B(1)</ul>
      | 
      | <p>The block inputs and output contain more than one signal as described below.</p>
      | 
      | <p><H4>Block Vector Input 1 - A</H4>
      | <ul>
      | <li>A(1)</li>
      | <li>A(2)</li>
      | <li>A(3)</li>
      | </ul>
      | </p>
      | 
      | <p><H4>Block Vector Input 2 - B</H4>
      | <ul>
      | <li>B(1)</li>
      | <li>B(2)</li>
      | <li>B(3)</li>
      | </ul>
      | </p>
      | 
      | <p><H4>Block Vector Output - Cross Product (AxB)</H4>
      | <ul>
      | <li>C(1)</li>
      | <li>C(2)</li>
      | <li>C(3)</li>
      | </ul>
      | </p>
      mask Display: disp('Cross\nProduct')
  Zeci x Reci1 : Subsystem  mask(Cross Product){}
      mask help: Calculates the cross product of two 3x1 vectors.
      mask Help:
      | <p>This block calculates the cross product of two 3x1 vectors, ie.</p>
      | 
      | <ul>C(1) = A(2)*B(3) - A(3)*B(2)</ul>
      | <ul>C(2) = A(3)*B(1) - A(1)*B(3)</ul>
      | <ul>C(3) = A(1)*B(2) - A(2)*B(1)</ul>
      | 
      | <p>The block inputs and output contain more than one signal as described below.</p>
      | 
      | <p><H4>Block Vector Input 1 - A</H4>
      | <ul>
      | <li>A(1)</li>
      | <li>A(2)</li>
      | <li>A(3)</li>
      | </ul>
      | </p>
      | 
      | <p><H4>Block Vector Input 2 - B</H4>
      | <ul>
      | <li>B(1)</li>
      | <li>B(2)</li>
      | <li>B(3)</li>
      | </ul>
      | </p>
      | 
      | <p><H4>Block Vector Output - Cross Product (AxB)</H4>
      | <ul>
      | <li>C(1)</li>
      | <li>C(2)</li>
      | <li>C(3)</li>
      | </ul>
      | </p>
      mask Display: disp('Cross\nProduct')
  yscbSCB : Constant  Value=[0 1 0]
  qscbp2scb : Outport
  wires:
  Direction Cosine Matrix to Quaternions/1 -> Quaternion Inverse/1  "qscbp2scb"
  Demux2/3 -> Create 3x3 Matrix/9
  Demux2/1 -> Create 3x3 Matrix/7
  Demux/1 -> Create 3x3 Matrix/1
  Demux1/2 -> Create 3x3 Matrix/5
  EORthrustSCB/1 -> VecNormalize4/1(In1)
  Demux2/2 -> Create 3x3 Matrix/8
  Demux/3 -> Create 3x3 Matrix/3
  Zeci x Reci/1(c(1) c(2) c(3)) -> Zeci x Reci1/2(b(1) b(2) b(3)), Demux/1  "xscbpSCB"
  Demux/2 -> Create 3x3 Matrix/2
  Create 3x3 Matrix/1 -> Direction Cosine Matrix to Quaternions/1
  Zeci x Reci1/1(c(1) c(2) c(3)) -> Demux1/1  "yscbpSCB"
  Demux1/3 -> Create 3x3 Matrix/6
  Demux1/1 -> Create 3x3 Matrix/4
  yscbSCB/1 -> Zeci x Reci/1(a(1) a(2) a(3))
  VecNormalize4/1(Out1) -> Demux2/1, Zeci x Reci1/1(a(1) a(2) a(3)), Zeci x Reci/2(b(1) b(2) b(3))  "zscbpSCB"
  Quaternion Inverse/1 -> qscbp2scb/1

== system HSat_orbit/Subsystem1/Subsystem4/EORattitude/Subsystem4/Subsystem1/q_scb_calc ==
  EORthrustECI : Inport
  sunvECI : Inport  Port=2
  Direction Cosine Matrix to Quaternions : sharedtransform/Direction Cosine Matrix  to Quaternions  aMode=0  action=None  tolerance=eps(2)
      settings: LibrarySourceBlock=|
      | aerolibtransform2/Direction Cosine Matrix
      | to Quaternions
  Matrix Concatenate : Concatenate  NumInputs=3  Mode=Multidimensional array
  Reshape1 : Reshape  OutputDimensionality=Row vector (2-D)
  Reshape2 : Reshape  OutputDimensionality=Row vector (2-D)
  Reshape3 : Reshape  OutputDimensionality=Row vector (2-D)
  VecNormalize : Subsystem
      mask Display: disp('u/||u||')
  VecNormalize1 : Subsystem
      mask Display: disp('u/||u||')
  VecNormalize2 : Subsystem
      mask Display: disp('u/||u||')
  VecNormalize3 : Subsystem
      mask Display: disp('u/||u||')
  Yscb x Zscb : Subsystem  mask(Cross Product){}
      mask help: Calculates the cross product of two 3x1 vectors.
      mask Help:
      | <p>This block calculates the cross product of two 3x1 vectors, ie.</p>
      | 
      | <ul>C(1) = A(2)*B(3) - A(3)*B(2)</ul>
      | <ul>C(2) = A(3)*B(1) - A(1)*B(3)</ul>
      | <ul>C(3) = A(1)*B(2) - A(2)*B(1)</ul>
      | 
      | <p>The block inputs and output contain more than one signal as described below.</p>
      | 
      | <p><H4>Block Vector Input 1 - A</H4>
      | <ul>
      | <li>A(1)</li>
      | <li>A(2)</li>
      | <li>A(3)</li>
      | </ul>
      | </p>
      | 
      | <p><H4>Block Vector Input 2 - B</H4>
      | <ul>
      | <li>B(1)</li>
      | <li>B(2)</li>
      | <li>B(3)</li>
      | </ul>
      | </p>
      | 
      | <p><H4>Block Vector Output - Cross Product (AxB)</H4>
      | <ul>
      | <li>C(1)</li>
      | <li>C(2)</li>
      | <li>C(3)</li>
      | </ul>
      | </p>
      mask Display: disp('Cross\nProduct')
  Zeci x Reci : Subsystem  mask(Cross Product){}
      mask help: Calculates the cross product of two 3x1 vectors.
      mask Help:
      | <p>This block calculates the cross product of two 3x1 vectors, ie.</p>
      | 
      | <ul>C(1) = A(2)*B(3) - A(3)*B(2)</ul>
      | <ul>C(2) = A(3)*B(1) - A(1)*B(3)</ul>
      | <ul>C(3) = A(1)*B(2) - A(2)*B(1)</ul>
      | 
      | <p>The block inputs and output contain more than one signal as described below.</p>
      | 
      | <p><H4>Block Vector Input 1 - A</H4>
      | <ul>
      | <li>A(1)</li>
      | <li>A(2)</li>
      | <li>A(3)</li>
      | </ul>
      | </p>
      | 
      | <p><H4>Block Vector Input 2 - B</H4>
      | <ul>
      | <li>B(1)</li>
      | <li>B(2)</li>
      | <li>B(3)</li>
      | </ul>
      | </p>
      | 
      | <p><H4>Block Vector Output - Cross Product (AxB)</H4>
      | <ul>
      | <li>C(1)</li>
      | <li>C(2)</li>
      | <li>C(3)</li>
      | </ul>
      | </p>
      mask Display: disp('Cross\nProduct')
  qECI2scbp : Outport  InitialOutput=0
  wires:
  Zeci x Reci/1(c(1) c(2) c(3)) -> VecNormalize3/1(In1)  "Y"
  VecNormalize1/1(Out1) -> Yscb x Zscb/2(b(1) b(2) b(3)), Reshape3/1, Zeci x Reci/2(b(1) b(2) b(3))  "Zscbp"
  Direction Cosine Matrix to Quaternions/1 -> qECI2scbp/1
  EORthrustECI/1 -> VecNormalize1/1(In1)
  VecNormalize3/1(Out1) -> Reshape1/1, Yscb x Zscb/1(a(1) a(2) a(3))  "Yscbp"
  Yscb x Zscb/1(c(1) c(2) c(3)) -> VecNormalize/1(In1)
  sunvECI/1 -> VecNormalize2/1(In1)
  Reshape1/1 -> Matrix Concatenate/2
  Reshape3/1 -> Matrix Concatenate/3
  Reshape2/1 -> Matrix Concatenate/1
  VecNormalize/1(Out1) -> Reshape2/1  "Xscbp"
  VecNormalize2/1(Out1) -> Zeci x Reci/1(a(1) a(2) a(3))
  Matrix Concatenate/1 -> Direction Cosine Matrix to Quaternions/1

== system HSat_orbit/Subsystem1/Subsystem4/EORattitude/Subsystem4/Subsystem2/VecNormalize4 ==
  In1 : Inport
  Constant : Constant
  Demux : Demux  Outputs=[-1 1]
  Divide : Product  Inputs=*/  OutDataTypeStr=double
  Ground : Ground
  Math Function : Math  Operator=square  SignedPower=on
  Math Function1 : Math  Operator=sqrt  SignedPower=on
  Mux : Mux  Inputs=2
  Mux1 : Mux  Inputs=2
  Product : Product  RndMeth=Zero
  Sum of Elements : Sum  Inputs=+
  Switch : Switch  Criteria=u2 > Threshold  Threshold=eps  SaturateOnIntegerOverflow=off  InputSameDT=off
  Out1 : Outport  VectorParamsAs1DForOutWhenUnconnected=off
  wires:
  Math Function/1 -> Sum of Elements/1
  Demux/1 -> Divide/1
  Constant/1 -> Mux1/2
  Mux1/1 -> Switch/3
  Divide/1 -> Out1/1
  Switch/1 -> Demux/1
  Mux/1 -> Switch/1
  Demux/2 -> Divide/2
  Product/1 -> Mux1/1
  In1/1 -> Product/1, Math Function/1, Mux/1
  Ground/1 -> Product/2
  Sum of Elements/1 -> Math Function1/1
  Math Function1/1 -> Mux/2, Switch/2

== system HSat_orbit/Subsystem1/Subsystem4/EORattitude/Subsystem4/Subsystem3/FlipSatellite ==
  AmomSCB : Inport
  EORtorqueSCB : Inport  Port=2
  Compare To Constant : simulink/Logic and Bit Operations/Compare To Constant  relop=>  const=sin((180-70.53)/2*pi/180)*25*.75  OutDataTypeStr=boolean
  Compare To Constant1 : simulink/Logic and Bit Operations/Compare To Constant  relop=>  const=cos(80*pi/180)  OutDataTypeStr=boolean
  Compare To Constant2 : simulink/Logic and Bit Operations/Compare To Constant  relop=>  const=sin((180-70.53)/2*pi/180)*25*.8  OutDataTypeStr=boolean
  Compare To Constant3 : simulink/Logic and Bit Operations/Compare To Constant  relop=>  const=cos(90*pi/180)  OutDataTypeStr=boolean
  Dot Product : DotProduct  OutDataTypeStr=Inherit: Inherit via internal rule
  Dot Product1 : DotProduct  OutDataTypeStr=Inherit: Inherit via internal rule
  Logical Operator : Logic  AllPortsSameDT=off  OutDataTypeStr=boolean
  Logical Operator1 : Logic  AllPortsSameDT=off  OutDataTypeStr=boolean
  Logical Operator2 : Logic  Operator=OR  AllPortsSameDT=off  OutDataTypeStr=boolean
  Logical Operator3 : Logic  Operator=NOT  AllPortsSameDT=off  OutDataTypeStr=boolean
  Reshape1 : Reshape  OutputDimensionality=Row vector (2-D)
  VecNormalize : Subsystem
      mask Display: disp('u/||u||')
  VecNormalize1 : Subsystem
      mask Display: disp('u/||u||')
  FlipSatellite_bool : Outport
  DoAMOM : Outport  Port=2
  NoAMOM : Outport  Port=3
  wires:
  Logical Operator/1 -> Logical Operator2/1
  EORtorqueSCB/1 -> VecNormalize1/1(In1)
  Dot Product/1 -> Compare To Constant2/1, Compare To Constant/1
  Compare To Constant/1 -> Logical Operator/1
  Dot Product1/1 -> Compare To Constant3/1, Compare To Constant1/1
  Compare To Constant1/1 -> Logical Operator/2
  VecNormalize/1(Out1) -> Dot Product/2, Dot Product1/1
  VecNormalize1/1(Out1) -> Dot Product1/2
  Compare To Constant2/1 -> Logical Operator1/1
  Compare To Constant3/1 -> Logical Operator3/1, Logical Operator1/2
  Logical Operator1/1 -> DoAMOM/1, Logical Operator2/2
  Logical Operator2/1 -> FlipSatellite_bool/1
  AmomSCB/1 -> Reshape1/1
  Reshape1/1 -> Dot Product/1, VecNormalize/1(In1)
  Logical Operator3/1 -> NoAMOM/1

== system HSat_orbit/Subsystem1/Subsystem4/EORattitude/Subsystem4/Subsystem3/Subsystem ==
  note: FlipSign
  FlipNow : Inport
  Logical Operator : Logic  Operator=NOT  AllPortsSameDT=off  OutDataTypeStr=boolean
  Switch : Switch  Criteria=u2 > Threshold  SaturateOnIntegerOverflow=off
  Unit Delay : UnitDelay  InitialCondition=false  SampleTime=-1  HasFrameUpgradeWarning=on
  FlipPlusMinus : Outport
  wires:
  FlipNow/1 -> Switch/2
  Logical Operator/1 -> Switch/1
  Switch/1 -> Unit Delay/1, FlipPlusMinus/1
  Unit Delay/1 -> Logical Operator/1, Switch/3

== system HSat_orbit/Subsystem1/Subsystem4/Subsystem6/Subsystem2/PPU1/VecNormalize1 ==
  In1 : Inport
  Constant : Constant
  Demux : Demux  Outputs=[-1 1]
  Divide : Product  Inputs=*/  OutDataTypeStr=double
  Ground : Ground
  Math Function : Math  Operator=square  SignedPower=on
  Math Function1 : Math  Operator=sqrt  SignedPower=on
  Mux : Mux  Inputs=2
  Mux1 : Mux  Inputs=2
  Product : Product  RndMeth=Zero
  Sum of Elements : Sum  Inputs=+
  Switch : Switch  Criteria=u2 > Threshold  Threshold=eps  SaturateOnIntegerOverflow=off  InputSameDT=off
  Out1 : Outport  VectorParamsAs1DForOutWhenUnconnected=off
  wires:
  Math Function/1 -> Sum of Elements/1
  Demux/1 -> Divide/1
  Constant/1 -> Mux1/2
  Mux1/1 -> Switch/3
  Divide/1 -> Out1/1
  Switch/1 -> Demux/1
  Mux/1 -> Switch/1
  Demux/2 -> Divide/2
  Product/1 -> Mux1/1
  In1/1 -> Product/1, Math Function/1, Mux/1
  Ground/1 -> Product/2
  Sum of Elements/1 -> Math Function1/1
  Math Function1/1 -> Mux/2, Switch/2

== system HSat_orbit/Subsystem1/Subsystem4/Subsystem6/Subsystem2/PPU1/VecNormalize2 ==
  In1 : Inport
  Constant : Constant
  Demux : Demux  Outputs=[-1 1]
  Divide : Product  Inputs=*/  OutDataTypeStr=double
  Ground : Ground
  Math Function : Math  Operator=square  SignedPower=on
  Math Function1 : Math  Operator=sqrt  SignedPower=on
  Mux : Mux  Inputs=2
  Mux1 : Mux  Inputs=2
  Product : Product  RndMeth=Zero
  Sum of Elements : Sum  Inputs=+
  Switch : Switch  Criteria=u2 > Threshold  Threshold=eps  SaturateOnIntegerOverflow=off  InputSameDT=off
  Out1 : Outport  VectorParamsAs1DForOutWhenUnconnected=off
  wires:
  Math Function/1 -> Sum of Elements/1
  Demux/1 -> Divide/1
  Constant/1 -> Mux1/2
  Mux1/1 -> Switch/3
  Divide/1 -> Out1/1
  Switch/1 -> Demux/1
  Mux/1 -> Switch/1
  Demux/2 -> Divide/2
  Product/1 -> Mux1/1
  In1/1 -> Product/1, Math Function/1, Mux/1
  Ground/1 -> Product/2
  Sum of Elements/1 -> Math Function1/1
  Math Function1/1 -> Mux/2, Switch/2

== system HSat_orbit/Subsystem1/Subsystem4/Subsystem6/Subsystem2/PPU1/VecNormalize3 ==
  In1 : Inport
  Constant : Constant
  Demux : Demux  Outputs=[-1 1]
  Divide : Product  Inputs=*/  OutDataTypeStr=double
  Ground : Ground
  Math Function : Math  Operator=square  SignedPower=on
  Math Function1 : Math  Operator=sqrt  SignedPower=on
  Mux : Mux  Inputs=2
  Mux1 : Mux  Inputs=2
  Product : Product  RndMeth=Zero
  Sum of Elements : Sum  Inputs=+
  Switch : Switch  Criteria=u2 > Threshold  Threshold=eps  SaturateOnIntegerOverflow=off  InputSameDT=off
  Out1 : Outport  VectorParamsAs1DForOutWhenUnconnected=off
  wires:
  Math Function/1 -> Sum of Elements/1
  Demux/1 -> Divide/1
  Constant/1 -> Mux1/2
  Mux1/1 -> Switch/3
  Divide/1 -> Out1/1
  Switch/1 -> Demux/1
  Mux/1 -> Switch/1
  Demux/2 -> Divide/2
  Product/1 -> Mux1/1
  In1/1 -> Product/1, Math Function/1, Mux/1
  Ground/1 -> Product/2
  Sum of Elements/1 -> Math Function1/1
  Math Function1/1 -> Mux/2, Switch/2

== system HSat_orbit/Subsystem1/Subsystem4/Subsystem6/Subsystem2/PPU1/VecNormalize4 ==
  In1 : Inport
  Constant : Constant
  Demux : Demux  Outputs=[-1 1]
  Divide : Product  Inputs=*/  OutDataTypeStr=double
  Ground : Ground
  Math Function : Math  Operator=square  SignedPower=on
  Math Function1 : Math  Operator=sqrt  SignedPower=on
  Mux : Mux  Inputs=2
  Mux1 : Mux  Inputs=2
  Product : Product  RndMeth=Zero
  Sum of Elements : Sum  Inputs=+
  Switch : Switch  Criteria=u2 > Threshold  Threshold=eps  SaturateOnIntegerOverflow=off  InputSameDT=off
  Out1 : Outport  VectorParamsAs1DForOutWhenUnconnected=off
  wires:
  Math Function/1 -> Sum of Elements/1
  Demux/1 -> Divide/1
  Constant/1 -> Mux1/2
  Mux1/1 -> Switch/3
  Divide/1 -> Out1/1
  Switch/1 -> Demux/1
  Mux/1 -> Switch/1
  Demux/2 -> Divide/2
  Product/1 -> Mux1/1
  In1/1 -> Product/1, Math Function/1, Mux/1
  Ground/1 -> Product/2
  Sum of Elements/1 -> Math Function1/1
  Math Function1/1 -> Mux/2, Switch/2

== system HSat_orbit/Subsystem1/Subsystem4/Subsystem6/Subsystem2/PPU1/VecNormalize5 ==
  In1 : Inport
  Constant : Constant
  Demux : Demux  Outputs=[-1 1]
  Divide : Product  Inputs=*/  OutDataTypeStr=double
  Ground : Ground
  Math Function : Math  Operator=square  SignedPower=on
  Math Function1 : Math  Operator=sqrt  SignedPower=on
  Mux : Mux  Inputs=2
  Mux1 : Mux  Inputs=2
  Product : Product  RndMeth=Zero
  Sum of Elements : Sum  Inputs=+
  Switch : Switch  Criteria=u2 > Threshold  Threshold=eps  SaturateOnIntegerOverflow=off  InputSameDT=off
  Out1 : Outport  VectorParamsAs1DForOutWhenUnconnected=off
  wires:
  Math Function/1 -> Sum of Elements/1
  Demux/1 -> Divide/1
  Constant/1 -> Mux1/2
  Mux1/1 -> Switch/3
  Divide/1 -> Out1/1
  Switch/1 -> Demux/1
  Mux/1 -> Switch/1
  Demux/2 -> Divide/2
  Product/1 -> Mux1/1
  In1/1 -> Product/1, Math Function/1, Mux/1
  Ground/1 -> Product/2
  Sum of Elements/1 -> Math Function1/1
  Math Function1/1 -> Mux/2, Switch/2

== system HSat_orbit/Subsystem1/Subsystem4/Subsystem6/Subsystem2/PPU1/VecNormalize6 ==
  In1 : Inport
  Constant : Constant
  Demux : Demux  Outputs=[-1 1]
  Divide : Product  Inputs=*/  OutDataTypeStr=double
  Ground : Ground
  Math Function : Math  Operator=square  SignedPower=on
  Math Function1 : Math  Operator=sqrt  SignedPower=on
  Mux : Mux  Inputs=2
  Mux1 : Mux  Inputs=2
  Product : Product  RndMeth=Zero
  Sum of Elements : Sum  Inputs=+
  Switch : Switch  Criteria=u2 > Threshold  Threshold=eps  SaturateOnIntegerOverflow=off  InputSameDT=off
  Out1 : Outport  VectorParamsAs1DForOutWhenUnconnected=off
  wires:
  Math Function/1 -> Sum of Elements/1
  Demux/1 -> Divide/1
  Constant/1 -> Mux1/2
  Mux1/1 -> Switch/3
  Divide/1 -> Out1/1
  Switch/1 -> Demux/1
  Mux/1 -> Switch/1
  Demux/2 -> Divide/2
  Product/1 -> Mux1/1
  In1/1 -> Product/1, Math Function/1, Mux/1
  Ground/1 -> Product/2
  Sum of Elements/1 -> Math Function1/1
  Math Function1/1 -> Mux/2, Switch/2

== system HSat_orbit/Subsystem1/Subsystem4/Subsystem6/Subsystem2/PPU1/VecNormalize7 ==
  In1 : Inport
  Constant : Constant
  Demux : Demux  Outputs=[-1 1]
  Divide : Product  Inputs=*/  OutDataTypeStr=double
  Ground : Ground
  Math Function : Math  Operator=square  SignedPower=on
  Math Function1 : Math  Operator=sqrt  SignedPower=on
  Mux : Mux  Inputs=2
  Mux1 : Mux  Inputs=2
  Product : Product  RndMeth=Zero
  Sum of Elements : Sum  Inputs=+
  Switch : Switch  Criteria=u2 > Threshold  Threshold=eps  SaturateOnIntegerOverflow=off  InputSameDT=off
  Out1 : Outport  VectorParamsAs1DForOutWhenUnconnected=off
  wires:
  Math Function/1 -> Sum of Elements/1
  Demux/1 -> Divide/1
  Constant/1 -> Mux1/2
  Mux1/1 -> Switch/3
  Divide/1 -> Out1/1
  Switch/1 -> Demux/1
  Mux/1 -> Switch/1
  Demux/2 -> Divide/2
  Product/1 -> Mux1/1
  In1/1 -> Product/1, Math Function/1, Mux/1
  Ground/1 -> Product/2
  Sum of Elements/1 -> Math Function1/1
  Math Function1/1 -> Mux/2, Switch/2

== system HSat_orbit/Subsystem1/Subsystem4/Subsystem6/Subsystem2/PPU1/VecNormalize8 ==
  In1 : Inport
  Constant : Constant
  Demux : Demux  Outputs=[-1 1]
  Divide : Product  Inputs=*/  OutDataTypeStr=double
  Ground : Ground
  Math Function : Math  Operator=square  SignedPower=on
  Math Function1 : Math  Operator=sqrt  SignedPower=on
  Mux : Mux  Inputs=2
  Mux1 : Mux  Inputs=2
  Product : Product  RndMeth=Zero
  Sum of Elements : Sum  Inputs=+
  Switch : Switch  Criteria=u2 > Threshold  Threshold=eps  SaturateOnIntegerOverflow=off  InputSameDT=off
  Out1 : Outport  VectorParamsAs1DForOutWhenUnconnected=off
  wires:
  Math Function/1 -> Sum of Elements/1
  Demux/1 -> Divide/1
  Constant/1 -> Mux1/2
  Mux1/1 -> Switch/3
  Divide/1 -> Out1/1
  Switch/1 -> Demux/1
  Mux/1 -> Switch/1
  Demux/2 -> Divide/2
  Product/1 -> Mux1/1
  In1/1 -> Product/1, Math Function/1, Mux/1
  Ground/1 -> Product/2
  Sum of Elements/1 -> Math Function1/1
  Math Function1/1 -> Mux/2, Switch/2
